simulink model "Islanding_case"  (R2024b)
settings: Solver=ode3  StartTime=0.0  StopTime=2.8  FixedStep=Ts  RelTol=1e-3  EnableMultiTasking=on
InitFcn:
  | Ts=100e-6;
  | Ts_Control=100e-6;
  | Ts_Power=100e-6;
  | tvv=0.1;
  | tr=1;
  | RelayEnableTime=1;
  | En_MC=1;
  | 
  | % ================= CHOOSE THE CASE HERE ==================
  | CaseNo    = 1;      % 1 = grid connected   2 = islanding   3 = fault during islanding
  | FaultType = 'none';   % 'none'  'LG'  'LL'  'LLG'  'LLL'  'LLLG'   (not used in case 2)
  | Qmismatch = 0;      % extra capacitive reactive power (% of 1.5 MW per load); try 1 in case 2 to see the inverter trip
  | % =========================================================
  | 
  | % ---- settings derived from the case (no need to edit)
  | switch CaseNo
  |     case 1, Tisland = 100; Pmismatch = 50; Tf = 2.0;   % grid + PV supply the load, fault at 2.0 s
  |     case 2, Tisland = 2.0; Pmismatch = 0;  Tf = 100;   % breakers open at 2.0 s, no fault
  |     case 3, Tisland = 2.0; Pmismatch = 0;  Tf = 2.3;   % breakers open at 2.0 s, fault at 2.3 s
  |     otherwise, error('CaseNo must be 1, 2 or 3');
  | end
  | FaultDur = 0.1;     % fault duration (s)
  | Tf_LG   = 100; Tf_LL = 100; Tf_LLG = 100; Tf_LLL = 100; Tf_LLLG = 100;   % 100 = never
  | switch upper(FaultType)
  |     case 'LG',   Tf_LG   = Tf;
  |     case 'LL',   Tf_LL   = Tf;
  |     case 'LLG',  Tf_LLG  = Tf;
  |     case 'LLL',  Tf_LLL  = Tf;
  |     case 'LLLG', Tf_LLLG = Tf;
  |     case 'NONE'
  |     otherwise, error('FaultType must be none, LG, LL, LLG, LLL or LLLG');
  | end
undefined symbols (not defined in the file or in its folder): DiscIntNeverNeededParam, Finit, Newton, Raphson, Tisland
libraries: simulink x33, spsOnDelayLib x17, powerlib_extras x11, eeGeneralControl x9, spsThreePhaseFaultLib x6, slpidlib x6, spsThreePhaseVIMeasurementLib x4, spsSampleandHoldLib x4, spsAlphaBetaZerotodq0Lib x4, spsThreePhaseSourceLib x4, spsThreePhaseBreakerLib x3, simulink_extras x3
(part 1 of 4)
settings Model: Creator=Administrator  LastModifiedBy=subas
settings SolverCC: AlgebraicLoopSolver=TrustRegion
settings DataIOCC: LimitDataPoints=on  SaveFormat=Array  SignalLoggingSaveFormat=ModelDataLogs  ReturnWorkspaceOutputs=off
settings OptimizationCC: ExpressionDepthLimit=2147483647  LifeSpan=inf
settings DebuggingCC: UnderspecifiedInitializationDetection=Classic  MergeDetectMultiDrivingBlocksExec=none  SolverPrmCheckMsg=warning  FcnCallInpInsideContextMsg=warning  UnconnectedInputMsg=warning  UnconnectedOutputMsg=warning  UnconnectedLineMsg=warning  StateNameClashWarn=warning  SFUnexpectedBacktrackingDiag=warning  SFNoUnconditionalDefaultTransitionDiag=warning  SFExecutionAtInitializationDiag=none  ArithmeticOperatorsInVariantConditions=warning
settings HardwareCC: ProdBitPerPointer=32  ProdBitPerSizeT=32  ProdBitPerPtrDiffT=32  ProdLargestAtomicFloat=None  ProdIntDivRoundTo=Undefined  ProdEndianess=Unspecified  ProdWordSize=32  ProdHWDeviceType=32-bit Generic
settings ModelReferenceCC: EnableRefExpFcnMdlSchedulingChecks=on  PropagateSignalLabelsOutOfModel=off
settings SFSimCC: SimUseLocalCustomCode=off  CustomCodeUndefinedFunction=UseInterfaceOnly
settings RTWCC: RTWUseLocalCustomCode=off  GPUComputeCapability=3.5
settings CodeAppCC: StateflowObjectComments=on
settings GRTTargetCC: TargetLangStandard=C89/C90 (ANSI)  CombineOutputUpdateFcns=off  GRTInterface=on
settings ConfigComp: CovMetricSettings=dw  CovSaveCumulativeToWorkspaceVar=on  CovSaveSingleToWorkspaceVar=on  CovExternalEMLEnable=off  CovSFcnEnable=off
settings SimscapeCC: SimscapeNormalizeSystem=off

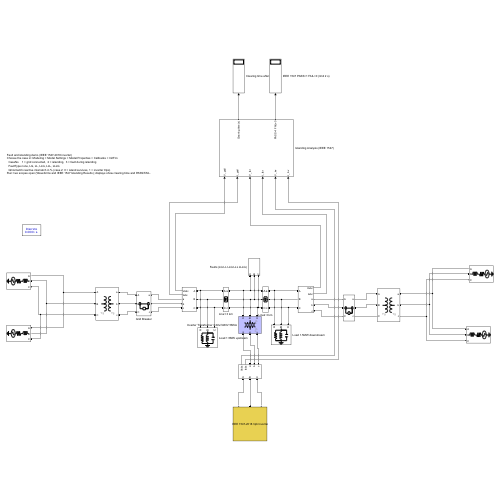
[thumbnail: Simulink's stored preview of the top-level diagram]
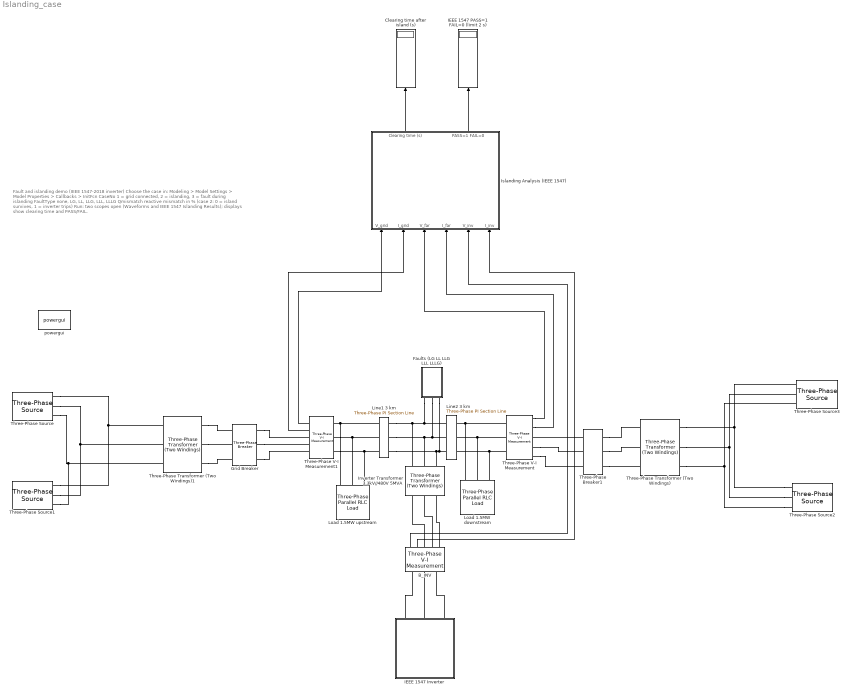
== system Islanding_case ==
  note: Fault and islanding demo (IEEE 1547-2018 inverter)
      | Choose the case in: Modeling > Model Settings > Model Properties > Callbacks > InitFcn
      |   CaseNo    1 = grid connected,  2 = islanding,  3 = fault during islanding
      |   FaultType none, LG, LL, LLG, LLL, LLLG
      |   Qmismatch reactive mismatch in % (case 2: 0 = island survives, 1 = inverter trips)
      | Run: two scopes open (Waveforms and IEEE 1547 Islanding Results); displays show clearing time and PASS/FAIL.
  B_INV : spsThreePhaseVIMeasurementLib/Three-Phase V-I Measurement  VoltageMeasurement=phase-to-ground  SetLabelV=off  LabelV=Vabc_PV  Vpu=off  VpuLL=off  CurrentMeasurement=yes  SetLabelI=off  LabelI=Iabc_PV  Ipu=off  Pbase=100e6  Vbase=500e3  OutputType=Complex  PhasorSimulation=off  PSBequivalent=0
  Clearing time after island (s) : Display
  Faults (LG LL LLG LLL LLLG) : Subsystem
  Grid Breaker : spsThreePhaseBreakerLib/Three-Phase Breaker  InitialState=closed  SwitchA=on  SwitchB=on  SwitchC=on  SwitchTimes=[Tisland]  External=off  BreakerResistance=0.001  SnubberResistance=1e6  SnubberCapacitance=inf  Measurements=None
  IEEE 1547 Inverter : Subsystem  mask(IEEE 1547-2018 Inverter){Pinv=1e6, N=3, RMSVnom=480/sqrt(3), NomFreq=50, Imax=1.2, Pref=1, EnableVW=0, En_VWatt=2, VWatt_V1=1.06, VWatt_V2=1.1, VWatt_P1=1, VWatt_P2=0, OLRT_VWatt=10, EnableFW=1, En_FW=2, dbOF=0.036, dbUF=0.036, KOF=0.05, KUF=0.05, Pmin=-1, OLRT_FW=5, EnableVQ=0, En_VVar=1, V1=0.92, V2=0.98, V3=1.02, V4=1.08, Q1=0.44, Q2=0, Q3=0, Q4=-0.44, OLRT_Vvar=5, QP_MODE_ENABLE=0, QP_CURVE_P1_GEN=0.2, QP_CURVE_P2_GEN=0.5, QP_CURVE_P3_GEN=1, QP_CURVE_Q1_GEN=0, QP_CURVE_Q2_GEN=0, QP_CURVE_Q3_GEN=-0.44, QP_CURVE_P1_ASP=-0.2, QP_CURVE_P2_ASP=-0.5, QP_CURVE_P3_ASP=-1, QP_CURVE_Q1_ASP=0, QP_CURVE_Q2_ASP=0, QP_CURVE_Q3_ASP=0.44, Constant_PF_Mode_Enable=0, Constant_PF=1, Constant_PF_Excitation=-1, CONST_Q_MODE_ENABLE=0, CONST_Q_ref=0, EnableMC=1, high_MC=1.2, low_MC=0.5, MC_recoveryrate=3, ES_V_HIGH=1.05, ES_V_LOW=0.917, ES_F_HIGH=50.1, ES_F_LOW=49.5, ES_DELAY=0, ES_RAMP_RATE=1, DVS_ENABLE=0, DVS_Threshold=0.88, Vref_DVS=1, Kpos=4, Kneg=4, EnableRMSOVProtection=1, OV2=1.2, OV2_time=0.16, OV1=1.1, OV1_time=13, UV1=0.88, UV1_time=21, UV2=0.5, UV2_time=2, EnableTOVProtection=1, EnableOFProtection=1, OF2=52, OF2_time=0.16, OF1=51.2, OF1_time=300, UF1=48.5, UF1_time=300, UF2=46.5, UF2_time=0.16, EnableOCProtection=1, OC2=2, OC2_time=0.16, OC1=1.5, OC1_time=0.5, GROUP2C_AI_ENABLE=1, GROUP2C_AI_DB=0.15, GROUP2C_AI_F_TH=2, GROUP2C_AI_LG1=0.1, GROUP2C_AI_LG2=0.2, GROUP2C_AI_HG1=0.2, GROUP2C_AI_HG2=0.2, GROUP2C_AI_LIMIT=0.5}
      mask prompts: Pinv "Inverter Apparent Power Rating (VA)"; N "Number of Inverters"; RMSVnom "Inverter Nominal RMS (l-g) Voltage (V)"; NomFreq "Nominal frequency (Hz)"; Imax "Maximum inverter current capacity (pu)"; Pref "Active Power reference (pu)"; EnableVW "Volt-Watt function Enable [Enable: 1; Disable: 0]"; En_VWatt "Enable Time Volt-Watt (sec)"; VWatt_V1 "VWatt curve point V1 setting (pu)"; VWatt_V2 "VWatt curve point V2 setting (pu)"; VWatt_P1 "VWatt curve point P1 setting (pu)"; VWatt_P2 "VWatt curve point P2 setting (pu)"; OLRT_VWatt "Open-Loop Response Time (sec)"; EnableFW "Freq-Watt function Enable [Enable: 1; Disable: 0]"; En_FW "Freq-Watt Enable Time (sec)"; dbOF "Over-freq deadband offset from nominal freq (Hz)"; dbUF "Under-freq deadband offset from nominal freq (Hz)"; KOF "Per unit over-freq change corresponding to a 1 pu power change"; KUF "Per unit under-freq change corresponding to a 1 pu power change"; Pmin "DER minimum active power (pu)"; OLRT_FW "Open-Loop Response Time (sec)"; EnableVQ "Volt-Var function Enable [Enable: 1; Disable: 0]"; En_VVar "Enable Time Volt-Var (sec)"; V1 "Voltage 1 (pu)"; V2 "Voltage 2 (pu)"; V3 "Voltage 3 (pu)"; V4 "Voltage 4 (pu)"; Q1 "Reactive Power 1 (pu)"; Q2 "Reactive Power 2 (pu)"; Q3 "Reactive Power 3 (pu)"; Q4 "Reactive Power 4 (pu)"; OLRT_Vvar "Open-Loop Response Time (sec)"; QP_MODE_ENABLE "Enable/Disable Watt-Var [Enable: 1; Diable: 0]"; QP_CURVE_P1_GEN "Watt-Var Curve Point P1 Setting (pu)"; QP_CURVE_P2_GEN "Watt-Var Curve Point P2 Setting (pu)"; QP_CURVE_P3_GEN "Watt-Var Curve Point P3 Setting (pu)"; QP_CURVE_Q1_GEN "Watt-Var Curve Point Q1 Setting (pu)"; QP_CURVE_Q2_GEN "Watt-Var Curve Point Q2 Setting (pu)"; QP_CURVE_Q3_GEN "Watt-Var Curve Point Q3 Setting (pu)"; QP_CURVE_P1_ASP "Watt-Var Curve Point P1' Setting (pu)"; QP_CURVE_P2_ASP "Watt-Var Curve Point P2' Setting (pu)"; QP_CURVE_P3_ASP "Watt-Var Curve Point P3' Setting (pu)"; QP_CURVE_Q1_ASP "Watt-Var Curve Point Q1' Setting (pu)"; QP_CURVE_Q2_ASP "Watt-Var Curve Point Q2' Setting (pu)"; QP_CURVE_Q3_ASP "Watt-Var Curve Point Q3' Setting (pu)"; Constant_PF_Mode_Enable "Enable/Disable Constant Power Factor [Enable: 1; Disable: 0]"; Constant_PF "Constant Power Factor Setting"; Constant_PF_Excitation "Constant Power Factor Excitation[Leading:1;Lagging:-1]"; CONST_Q_MODE_ENABLE "Enable/Disable Constant Reactive Power [Enable: 1; Disable: 0]"; CONST_Q_ref "Enter Reactive Power Reference Using the External Input [Injection:Positive;Absorption:Negative]"; EnableMC "Momentary Cessation Enable [Enable: 1; Disable: 0]"; high_MC "High-voltage momentary cessation threshold (pu)"; low_MC "Low-voltage momentary cessation threshold (pu)"; MC_recoveryrate "Momentary cessation recovery rate (pu/sec)"; ES_V_HIGH "Maximum applicable voltage to enter service (pu)"; ES_V_LOW "Minimum applicable voltage to enter service (pu)"; ES_F_HIGH "Maximum frequency to enter service (Hz)"; ES_F_LOW "Minimum frequency to enter service (Hz)"; ES_DELAY "Intentional delay before initiating soft-start (s)"; ES_RAMP_RATE "Enter active power ramp rate (pu/s)"; DVS_ENABLE "Enable/Disable DVS [Enable: 1; Disable: 0]"; DVS_Threshold "Voltage Threshold"; Vref_DVS "Pos seq Vref"; Kpos "Pos seq Kcomp"; Kneg "Neg seq Kcomp"; EnableRMSOVProtection "Enable/Disable RMS-based under- and over-voltage protection [Enable:1; Disable:0]"; OV2 "High voltage must trip OV2 voltage setting (pu)"; OV2_time "High voltage must trip OV2 duration setting (sec)"; OV1 "High voltage must trip OV1 voltage setting (pu)"; OV1_time "High voltage must trip OV1 duration setting (sec)"; UV1 "Low voltage must trip UV1 voltage setting (pu)"; UV1_time "Low voltage must trip UV1 duration setting (sec)"; UV2 "Low voltage must trip UV2 voltage setting (pu)"; UV2_time "Low voltage must trip UV2 duration setting (sec)"; EnableTOVProtection "Enable/Disable protection [Enable:1; Disable:0]"; EnableOFProtection "Enable/Disable under- and over-freqeuncy protection [Enable:1; Disable:0]"; OF2 "High freq must trip OF2 freq setting (Hz)"; OF2_time "High freq must trip OF2 duration setting (sec)"; OF1 "High freq must trip OF1 freq setting (Hz)"; OF1_time "High freq must trip OF1 duration setting (sec)"; UF1 "Low freq must trip UF1 freq setting (Hz)"; UF1_time "Low freq must trip UF1 duration setting (sec)"; UF2 "Low freq must trip UF2 freq setting (Hz)"; UF2_time "Low freq must trip UF2 duration setting (sec)"; EnableOCProtection "Enable/Disable under- and over-current protection [Enable:1; Disable:0]"; OC2 "Over-current must trip curve point OC2 current setting (pu)"; OC2_time "Over-current must trip curve point OC2 duration setting (s)"; OC1 "Over-current must trip curve point OC1 current setting (pu)"; OC1_time "Over-current must trip curve point OC1 duration setting (s)"; GROUP2C_AI_ENABLE "Enable/Disable Active Islanding Detection [Enable: 1; Disable: 0]"; GROUP2C_AI_DB "Dead-Band (No perturbations within deadband)"; GROUP2C_AI_F_TH "Frequency Threshold (Hz)"; GROUP2C_AI_LG1 "Low frequency gain 1"; GROUP2C_AI_LG2 "Low frequency gain 2"; GROUP2C_AI_HG1 "High frequency gain 1"; GROUP2C_AI_HG2 "High frequency gain 2"; GROUP2C_AI_LIMIT "Limit on reactive power perturbations (pu)"
      mask help:
      | Note:
      |  1) The active power rating (Watt) and the apparent power rating (VA) are the same for this inverter
      |  2) Any disturbances (fault, etc.) should be applied after the startup process has completed and a steady state has been reached
      |  3) Make sure ONLY ONE Reactive Power Support Function is activated (Volt-Var, Constant PF, Constant Q, or Watt-Var)
      |  4) Enable times for Volt-Watt, Volt-Var, and Freq-Watt functions are not inverter settings but provided to allow a user to simulate the impact of activating these functions
      |  5) When representing a battery or PV plus battery inverter:
      |    a) The active power reference should be set to a negative value (between -1pu and 0) if the inverter is in charging mode
      |    b) The Volt-Watt curve point P2 and the Freq-Watt DER minimum active power settings can be set to negative values between -1pu and 0
      mask DialogControl ParameterTabVar01 Prompt: Physical Elements
      mask DialogControl Container17 Prompt: Control Elements
      mask DialogControl Container31 Prompt: Active Power Support Functions
      mask DialogControl Container54 Prompt: 1. Voltage-Active Power (Volt-Watt) Function
      mask DialogControl Container32 Prompt: 2. Frequency - Active Power (Frequency-Watt) Function
      mask DialogControl Container37 Prompt: Reactive Power Support Functions
      mask DialogControl Container38 Prompt: 1. Voltage-Reactive Power (Volt-Var) Function
      mask DialogControl Container40 Prompt: 2. Active Power-Reactive Power (Watt - Var) Function
      mask DialogControl Container42 Prompt: 3. Constant Power Factor Function
      mask DialogControl Container44 Prompt: 4. Constant Reactive Power Mode
      mask DialogControl Container46 Prompt: Momentary Cessation
      mask DialogControl Container48 Prompt: Enter Service Criteria
      mask DialogControl Container53 Prompt: Dynamic Voltage Support
      mask DialogControl Container26 Prompt: Protection Elements
      mask DialogControl Container20 Prompt: Under- and Over-voltage protection
      mask DialogControl Container56 Prompt: Transient Over-Voltage Protection
      mask DialogControl Container22 Prompt: Under-and Over-frequency protection
      mask DialogControl Container24 Prompt: Over Current Protection
      mask DialogControl Container50 Prompt: Active Islanding Detection
      mask Display: disp('IEEE 1547-2018 3ph Inverter')
  IEEE 1547 PASS=1 FAIL=0 (limit 2 s) : Display
  Inverter Transformer 3.3kV//480V 5MVA : spsThreePhaseTransformerTwoWindingsLib/Three-Phase Transformer (Two Windings)  Winding1Connection=Yg  Winding2Connection=Yg  CoreType=Three single-phase transformers  SetSaturation=off  Hysteresis=off  DataFile='basic_model'  SetInitialFlux=off  Measurements=None  UNITS=pu  NominalPower=[5e6 50]  Winding1="[ 3.3e3  0.025/10   0.025 ]"  Winding2="[ 480  0.025/10  0.025]"  Rm=500  Lm=500  L0=0.5  Saturation="[ 0,0  ;  0.005,1.2  ;  1.0,1.4 ]"  InitialFluxes=[ 0.8 , -0.8 , 0.7 ]  BreakLoop=off  DiscreteSolver=Trapezoidal iterative  DataType=off  TransfoNumber=0
  Islanding Analysis (IEEE 1547) : Subsystem
  Line1 3 km : spsThreePhasePISectionLineLib/Three-Phase PI Section Line  LConnTagsString=a|b|c  RConnTagsString=A|B|C  Length=3  Frequency=50  Resistances=[0.0132 0.132]  Inductances=[0.9337e-3 4.1264e-3]  Capacitances=[12.74e-9 7.751e-9]
  Line2 3 km : spsThreePhasePISectionLineLib/Three-Phase PI Section Line  LConnTagsString=a|b|c  RConnTagsString=A|B|C  Length=3  Frequency=50  Resistances=[0.0132 0.132]  Inductances=[0.9337e-3 4.1264e-3]  Capacitances=[12.74e-9 7.751e-9]
  Load 1.5MW downstream : spsThreePhaseParallelRLCLoadLib/Three-Phase Parallel RLC Load  LConnTagsString=A|B|C  Configuration=Y (grounded)  NominalVoltage=3.3e3  Vabc=[1e3 1e3 1e3]  Vabcp=[1e3 1e3 1e3]  NominalFrequency=50  UnbalancedPower=off  ActivePower=1.48367e+06*(1+Pmismatch/100)  InductivePower=1.37206e+06  CapacitivePower=1.60436e+06+Qmismatch/100*1.5e6  Pabc=[10e3 9e3 11e3]  QLabc=[100 90 110]  QCabc=[100 90 110]  Pabcp=[10e3 9e3 11e3]  QLabcp=[100 90 110]  QCabcp=[100 90 110]  Measurements=None  LoadType=constant Z
  Load 1.5MW upstream : spsThreePhaseParallelRLCLoadLib/Three-Phase Parallel RLC Load  LConnTagsString=A|B|C  Configuration=Y (grounded)  NominalVoltage=3.3e3  Vabc=[1e3 1e3 1e3]  Vabcp=[1e3 1e3 1e3]  NominalFrequency=50  UnbalancedPower=off  ActivePower=1.48335e+06*(1+Pmismatch/100)  InductivePower=1.37193e+06  CapacitivePower=1.60383e+06+Qmismatch/100*1.5e6  Pabc=[10e3 9e3 11e3]  QLabc=[100 90 110]  QCabc=[100 90 110]  Pabcp=[10e3 9e3 11e3]  QLabcp=[100 90 110]  QCabcp=[100 90 110]  Measurements=None  LoadType=constant Z
  Three-Phase Transformer (Two Windings)1 : spsThreePhaseTransformerTwoWindingsLib/Three-Phase Transformer (Two Windings)  Winding1Connection=Yg  Winding2Connection=Yg  CoreType=Three single-phase transformers  SetSaturation=off  Hysteresis=off  DataFile='hysteresis'  SetInitialFlux=off  Measurements=None  UNITS=pu  NominalPower=[ 250e6 , 50 ]  Winding1=[132e3 , 0.002 , 0.08 ]  Winding2=[3.3e3 , 0.002 , 0.08 ]  Rm=500  Lm=500  L0=0.5  Saturation=[ 0,0 ; 0.0024,1.2 ; 1.0,1.52 ]  InitialFluxes=[ 0.8 , -0.8 , 0.7 ]  BreakLoop=off  DiscreteSolver=Trapezoidal iterative  DataType=off  TransfoNumber=1
  Three-Phase V-I Measurement : spsThreePhaseVIMeasurementLib/Three-Phase V-I Measurement  VoltageMeasurement=phase-to-ground  SetLabelV=off  LabelV=Vabc  Vpu=off  VpuLL=off  CurrentMeasurement=yes  SetLabelI=off  LabelI=Iabc  Ipu=off  Pbase=100e6  Vbase=500e3  OutputType=Complex  PhasorSimulation=off  PSBequivalent=0
  Three-Phase V-I Measurement1 : spsThreePhaseVIMeasurementLib/Three-Phase V-I Measurement  VoltageMeasurement=phase-to-ground  SetLabelV=off  LabelV=Vabc  Vpu=off  VpuLL=off  CurrentMeasurement=yes  SetLabelI=off  LabelI=Iabc  Ipu=off  Pbase=100e6  Vbase=500e3  OutputType=Complex  PhasorSimulation=off  PSBequivalent=0
  Three-Phase Breaker1 : spsThreePhaseBreakerLib/Three-Phase Breaker  InitialState=closed  SwitchA=on  SwitchB=on  SwitchC=on  SwitchTimes=[Tisland]  External=off  BreakerResistance=0.001  SnubberResistance=1e6  SnubberCapacitance=inf  Measurements=None
  Three-Phase Source : spsThreePhaseSourceLib/Three-Phase Source  InternalConnection=Yg  VoltagePhases=off  Voltage=132e3  PhaseAngle=0  Voltage_phases=[25e3 25e3 25e3]/sqrt(3)  PhaseAngles_phases=[0 -120 +120]  Frequency=50  NonIdealSource=on  SpecifyImpedance=off  Resistance=12  Inductance=16.58e-3  ShortCircuitLevel=50e6  BaseVoltage=11e3  XRratio=7  BusType=PV  Pref=50e6  Qref=0  Prefabc=[10e3, 10e3, 10e3]  Qrefabc=[0, 0, 0]  Qmin=-inf  Qmax=inf
  Three-Phase Source1 : spsThreePhaseSourceLib/Three-Phase Source  InternalConnection=Yg  VoltagePhases=off  Voltage=132e3  PhaseAngle=0  Voltage_phases=[25e3 25e3 25e3]/sqrt(3)  PhaseAngles_phases=[0 -120 +120]  Frequency=50  NonIdealSource=on  SpecifyImpedance=off  Resistance=12  Inductance=16.58e-3  ShortCircuitLevel=50e6  BaseVoltage=11e3  XRratio=7  BusType=PV  Pref=50e6  Qref=0  Prefabc=[10e3, 10e3, 10e3]  Qrefabc=[0, 0, 0]  Qmin=-inf  Qmax=inf
  Three-Phase Source2 : spsThreePhaseSourceLib/Three-Phase Source  InternalConnection=Yg  VoltagePhases=off  Voltage=132e3  PhaseAngle=0  Voltage_phases=[25e3 25e3 25e3]/sqrt(3)  PhaseAngles_phases=[0 -120 +120]  Frequency=50  NonIdealSource=on  SpecifyImpedance=off  Resistance=8.4  Inductance=16.58e-3  ShortCircuitLevel=20e6  BaseVoltage=11e3  XRratio=7  BusType=PV  Pref=20e6  Qref=0  Prefabc=[10e3, 10e3, 10e3]  Qrefabc=[0, 0, 0]  Qmin=-inf  Qmax=inf
  Three-Phase Source3 : spsThreePhaseSourceLib/Three-Phase Source  InternalConnection=Yg  VoltagePhases=off  Voltage=132e3  PhaseAngle=0  Voltage_phases=[25e3 25e3 25e3]/sqrt(3)  PhaseAngles_phases=[0 -120 +120]  Frequency=50  NonIdealSource=on  SpecifyImpedance=off  Resistance=12  Inductance=16.58e-3  ShortCircuitLevel=50e6  BaseVoltage=11e3  XRratio=7  BusType=PV  Pref=50e6  Qref=0  Prefabc=[10e3, 10e3, 10e3]  Qrefabc=[0, 0, 0]  Qmin=-inf  Qmax=inf
  Three-Phase Transformer (Two Windings) : spsThreePhaseTransformerTwoWindingsLib/Three-Phase Transformer (Two Windings)  Winding1Connection=Yg  Winding2Connection=Yg  CoreType=Three single-phase transformers  SetSaturation=off  Hysteresis=off  DataFile='hysteresis'  SetInitialFlux=off  Measurements=None  UNITS=pu  NominalPower=[ 250e6 , 50 ]  Winding1=[3.3e3 , 0.002 , 0.08 ]  Winding2=[132e3 , 0.002 , 0.08 ]  Rm=500  Lm=500  L0=0.5  Saturation=[ 0,0 ; 0.0024,1.2 ; 1.0,1.52 ]  InitialFluxes=[ 0.8 , -0.8 , 0.7 ]  BreakLoop=off  DiscreteSolver=Trapezoidal iterative  DataType=off  TransfoNumber=1
  powergui : spspowerguiLib/powergui  Priority=1  SimulationMode=Discrete  SampleTime=Ts  frequency=50  Iterations=50  frequencyindice=50  Pbase=100e6  ErrMax=1e-4  UnitsV=kV  UnitsW=MW  buscounter=0  FunctionMessages=off  echomessages=off  EnableUseOfTLC=off  CurrentSourceSwitches=off  DisableSnubberDevices=off  DisableRonSwitches=off  DisableVfSwitches=off  DisplayEquations=off  AutomaticDiscreteSolvers=off  SolverType=Tustin  Interpol=off  ExternalGateDelay=off  methode=off  Ts=0  x0status=blocks  SPID=off  SwTol=0  HookPort=off  NonlinearTolerance=1e-4  nMaxIteration=100  ContinueOnMaxIteration=off  RestoreLinks=warning  ResistiveCurrentMeasurement=off  Frange=[0:2:500]  Ylog=off  Xlog=on  ShowGrid=off  save=off  variable=ZData  structure=0  ZoomFFT=off  StartTime=0.0  cycles=1  DisplayStyle=1  fundamental=60  FreqAxis=off  MaxFrequency=1000  frequencyindicesteady=1  RmsSteady=1  display=off
  wires:
  Three-Phase V-I Measurement1/1 -> Islanding Analysis (IEEE 1547)/1(V_grid)
  Three-Phase V-I Measurement1/2 -> Islanding Analysis (IEEE 1547)/2(I_grid)
  Three-Phase V-I Measurement/1 -> Islanding Analysis (IEEE 1547)/3(V_far)
  Three-Phase V-I Measurement/2 -> Islanding Analysis (IEEE 1547)/4(I_far)
  B_INV/1 -> Islanding Analysis (IEEE 1547)/5(V_inv)
  B_INV/2 -> Islanding Analysis (IEEE 1547)/6(I_inv)
  Islanding Analysis (IEEE 1547)/1(Clearing time (s)) -> Clearing time after island (s)/1
  Islanding Analysis (IEEE 1547)/2(PASS=1 FAIL=0) -> IEEE 1547 PASS=1 FAIL=0 (limit 2 s)/1
  connections:
  Line1 3 km/RConn1 -- Inverter Transformer 3.3kV//480V 5MVA/LConn1 -- Faults (LG LL LLG LLL LLLG)/LConn1 -- Line2 3 km/LConn1
  Line1 3 km/RConn3 -- Inverter Transformer 3.3kV//480V 5MVA/LConn3 -- Faults (LG LL LLG LLL LLLG)/LConn3 -- Line2 3 km/LConn3
  Line1 3 km/RConn2 -- Inverter Transformer 3.3kV//480V 5MVA/LConn2 -- Faults (LG LL LLG LLL LLLG)/LConn2 -- Line2 3 km/LConn2
  Three-Phase Source/RConn1 -- Three-Phase Source1/RConn1 -- Three-Phase Transformer (Two Windings)1/LConn1
  Three-Phase Source/RConn2 -- Three-Phase Source1/RConn2 -- Three-Phase Transformer (Two Windings)1/LConn2
  Three-Phase Source/RConn3 -- Three-Phase Source1/RConn3 -- Three-Phase Transformer (Two Windings)1/LConn3
  Three-Phase V-I Measurement1/LConn1 -- Line1 3 km/LConn1 -- Load 1.5MW upstream/LConn1
  Three-Phase V-I Measurement1/LConn2 -- Line1 3 km/LConn2 -- Load 1.5MW upstream/LConn2
  Three-Phase V-I Measurement1/LConn3 -- Line1 3 km/LConn3 -- Load 1.5MW upstream/LConn3
  Line2 3 km/RConn1 -- Three-Phase V-I Measurement/LConn1 -- Load 1.5MW downstream/LConn1
  Line2 3 km/RConn2 -- Three-Phase V-I Measurement/LConn2 -- Load 1.5MW downstream/LConn2
  Line2 3 km/RConn3 -- Three-Phase V-I Measurement/LConn3 -- Load 1.5MW downstream/LConn3
  IEEE 1547 Inverter/LConn1 -- B_INV/LConn1
  B_INV/RConn1 -- Inverter Transformer 3.3kV//480V 5MVA/RConn1
  IEEE 1547 Inverter/LConn2 -- B_INV/LConn2
  B_INV/RConn2 -- Inverter Transformer 3.3kV//480V 5MVA/RConn2
  IEEE 1547 Inverter/LConn3 -- B_INV/LConn3
  B_INV/RConn3 -- Inverter Transformer 3.3kV//480V 5MVA/RConn3
  Three-Phase Source2/RConn1 -- Three-Phase Transformer (Two Windings)/RConn1 -- Three-Phase Source3/RConn1
  Three-Phase Source2/RConn2 -- Three-Phase Transformer (Two Windings)/RConn2 -- Three-Phase Source3/RConn2
  Three-Phase Source2/RConn3 -- Three-Phase Transformer (Two Windings)/RConn3 -- Three-Phase Source3/RConn3
  Three-Phase Transformer (Two Windings)1/RConn1 -- Grid Breaker/LConn1
  Grid Breaker/RConn1 -- Three-Phase V-I Measurement1/RConn1
  Three-Phase Transformer (Two Windings)1/RConn2 -- Grid Breaker/LConn2
  Grid Breaker/RConn2 -- Three-Phase V-I Measurement1/RConn2
  Three-Phase Transformer (Two Windings)1/RConn3 -- Grid Breaker/LConn3
  Grid Breaker/RConn3 -- Three-Phase V-I Measurement1/RConn3
  Three-Phase Breaker1/LConn1 -- Three-Phase V-I Measurement/RConn1
  Three-Phase Breaker1/RConn1 -- Three-Phase Transformer (Two Windings)/LConn1
  Three-Phase V-I Measurement/RConn2 -- Three-Phase Breaker1/LConn2
  Three-Phase Breaker1/RConn2 -- Three-Phase Transformer (Two Windings)/LConn2
  Three-Phase V-I Measurement/RConn3 -- Three-Phase Breaker1/LConn3
  Three-Phase Breaker1/RConn3 -- Three-Phase Transformer (Two Windings)/LConn3

== system Islanding_case/Faults (LG LL LLG LLL LLLG) ==
  Three-Phase Fault1 : spsThreePhaseFaultLib/Three-Phase Fault  InitialStates=0  FaultA=on  FaultB=on  FaultC=off  GroundFault=on  SwitchTimes=[Tf_LLG Tf_LLG+FaultDur]  External=off  SwitchStatus=NaN  FaultResistance=0.001  GroundResistance=0.001  SnubberResistance=1e6  SnubberCapacitance=inf  Measurements=None
  Three-Phase Fault2 : spsThreePhaseFaultLib/Three-Phase Fault  InitialStates=0  FaultA=on  FaultB=off  FaultC=off  GroundFault=on  SwitchTimes=[Tf_LG Tf_LG+FaultDur]  External=off  SwitchStatus=NaN  FaultResistance=0.001  GroundResistance=0.001  SnubberResistance=1e6  SnubberCapacitance=inf  Measurements=None
  Three-Phase Fault3 : spsThreePhaseFaultLib/Three-Phase Fault  InitialStates=0  FaultA=off  FaultB=on  FaultC=on  GroundFault=off  SwitchTimes=[Tf_LL Tf_LL+FaultDur]  External=off  SwitchStatus=NaN  FaultResistance=0.001  GroundResistance=0.001  SnubberResistance=1e6  SnubberCapacitance=inf  Measurements=None
  Three-Phase Fault4 : spsThreePhaseFaultLib/Three-Phase Fault  InitialStates=0  FaultA=on  FaultB=on  FaultC=on  GroundFault=on  SwitchTimes=[Tf_LLLG Tf_LLLG+FaultDur]  External=off  SwitchStatus=NaN  FaultResistance=0.001  GroundResistance=0.001  SnubberResistance=1e6  SnubberCapacitance=inf  Measurements=None
  Three-Phase Fault5 : spsThreePhaseFaultLib/Three-Phase Fault  InitialStates=0  FaultA=on  FaultB=on  FaultC=on  GroundFault=off  SwitchTimes=[Tf_LLL Tf_LLL+FaultDur]  External=off  SwitchStatus=NaN  FaultResistance=0.001  GroundResistance=0.001  SnubberResistance=1e6  SnubberCapacitance=inf  Measurements=None
  Three-Phase Fault6 : spsThreePhaseFaultLib/Three-Phase Fault  InitialStates=0  FaultA=off  FaultB=off  FaultC=off  GroundFault=off  SwitchTimes=[100 100.05]  External=off  SwitchStatus=NaN  FaultResistance=0.001  GroundResistance=0.001  SnubberResistance=1e6  SnubberCapacitance=inf  Measurements=None
  A : PMIOPort  Side=Left
  B : PMIOPort  Port=2  Side=Left
  C : PMIOPort  Port=3  Side=Left
  connections:
  Three-Phase Fault2/LConn2 -- Three-Phase Fault6/LConn2 -- Three-Phase Fault4/LConn2 -- Three-Phase Fault5/LConn2 -- Three-Phase Fault3/LConn2 -- Three-Phase Fault1/LConn2 -- B/RConn1
  Three-Phase Fault2/LConn3 -- Three-Phase Fault6/LConn3 -- Three-Phase Fault4/LConn3 -- Three-Phase Fault5/LConn3 -- Three-Phase Fault3/LConn3 -- Three-Phase Fault1/LConn3 -- C/RConn1
  Three-Phase Fault2/LConn1 -- Three-Phase Fault6/LConn1 -- Three-Phase Fault4/LConn1 -- Three-Phase Fault5/LConn1 -- Three-Phase Fault3/LConn1 -- Three-Phase Fault1/LConn1 -- A/RConn1

== system Islanding_case/IEEE 1547 Inverter ==
  " Inverter Hardware" : Subsystem
  DC Voltage Source : spsDCVoltageSourceLib/DC Voltage Source  Amplitude=RMSVnom*sqrt(3)*2.5  Measurements=None
  "Inverter measurements, controls, and protection" : Subsystem
  A : PMIOPort  Tag=PMCPort  Side=Left
  B : PMIOPort  Tag=PMCPort  Port=2  Side=Left
  C : PMIOPort  Tag=PMCPort  Port=3  Side=Left
  wires:
  [AC_Brk_Ctrl] -> " Inverter Hardware"/2(AC_Brk_Ctrl)
  [Uref] -> " Inverter Hardware"/1(Uref)
  [VPCC] -> "Inverter measurements, controls, and protection"/1(VPCC_inv)
  "Inverter measurements, controls, and protection"/1(Uref) -> [Uref]
  "Inverter measurements, controls, and protection"/2(AC Brk Ctrl) -> [AC_Brk_Ctrl]
  [IPCC] -> "Inverter measurements, controls, and protection"/2(IPCC)
  " Inverter Hardware"/2(IPCC) -> [IPCC]
  " Inverter Hardware"/1(VPCC) -> [VPCC]
  connections:
  DC Voltage Source/LConn1 -- " Inverter Hardware"/LConn2
  DC Voltage Source/RConn1 -- " Inverter Hardware"/LConn1
  " Inverter Hardware"/RConn3 -- C/RConn1
  " Inverter Hardware"/RConn2 -- B/RConn1
  " Inverter Hardware"/RConn1 -- A/RConn1

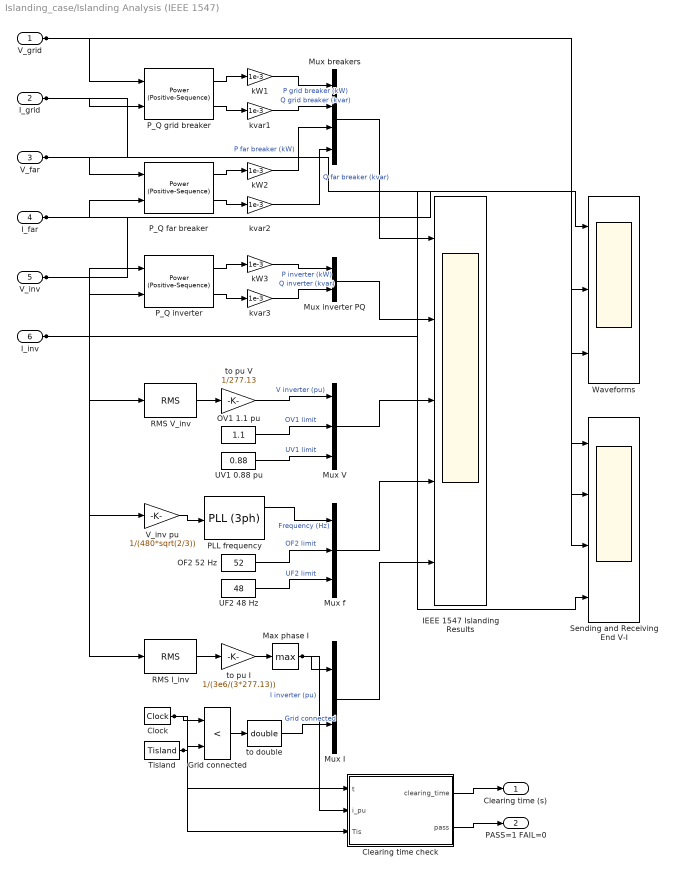
== system Islanding_case/Islanding Analysis (IEEE 1547) ==
  V_grid : Inport
  I_grid : Inport  Port=2
  V_far : Inport  Port=3
  I_far : Inport  Port=4
  V_inv : Inport  Port=5
  I_inv : Inport  Port=6
  Clearing time check : MATLAB Function  TreatAsAtomicUnit=on
  Clock : DigitalClock  SampleTime=Ts
  Grid connected : RelationalOperator  Operator=<  OutDataTypeStr=boolean  RndMeth=Simplest  InputSameDT=off
  IEEE 1547 Islanding Results : Scope  NumInputPorts=5
  Max phase I : MinMax  Function=max
  Mux I : Mux  Inputs=2
  Mux V : Mux  Inputs=3
  Mux breakers : Mux
  Mux f : Mux  Inputs=3
  Mux inverter PQ : Mux  Inputs=2
  OF2 52 Hz : Constant  Value=52  SampleTime=Ts
  OV1 1.1 pu : Constant  Value=1.1  SampleTime=Ts
  PLL frequency : spsPLL3phLib/PLL (3ph)  Fmin=40  Par_Init=[0, 50]  ParK=[180, 3200, 1]  TcD=1e-4  MaxRateChangeFreq=200  FilterCutOffFreq=25  Ts=Ts  AGC=on
  P_Q far breaker : spsPowerPositiveSequenceLib/Power (Positive-Sequence)  Freq=50  Vinit=[0, 0]  Iinit=[0, 0]  Ts=Ts
  P_Q grid breaker : spsPowerPositiveSequenceLib/Power (Positive-Sequence)  Freq=50  Vinit=[0, 0]  Iinit=[0, 0]  Ts=Ts
  P_Q inverter : spsPowerPositiveSequenceLib/Power (Positive-Sequence)  Freq=50  Vinit=[0, 0]  Iinit=[0, 0]  Ts=Ts
  RMS I_inv : spsRMSLib/RMS  TrueRMS=on  Freq=50  RMSInit=0  Ts=Ts
  RMS V_inv : spsRMSLib/RMS  TrueRMS=on  Freq=50  RMSInit=277.13  Ts=Ts
  Sending and Receiving End V-I : Scope  NumInputPorts=4
  Tisland : Constant  Value=Tisland  SampleTime=Ts
  UF2 48 Hz : Constant  Value=48  SampleTime=Ts
  UV1 0.88 pu : Constant  Value=0.88  SampleTime=Ts
  V_inv pu : Gain  Gain=1/(480*sqrt(2/3))
  Waveforms : Scope  NumInputPorts=3
  kW1 : Gain  Gain=1e-3
  kW2 : Gain  Gain=1e-3
  kW3 : Gain  Gain=1e-3
  kvar1 : Gain  Gain=1e-3
  kvar2 : Gain  Gain=1e-3
  kvar3 : Gain  Gain=1e-3
  to double : DataTypeConversion  OutDataTypeStr=double  SaturateOnIntegerOverflow=off  RndMeth=Floor
  to pu I : Gain  Gain=1/(3e6/(3*277.13))
  to pu V : Gain  Gain=1/277.13
  Clearing time (s) : Outport
  PASS=1 FAIL=0 : Outport  Port=2
  wires:
  V_grid/1 -> P_Q grid breaker/1, Sending and Receiving End V-I/1
  I_grid/1 -> P_Q grid breaker/2, Waveforms/1, Sending and Receiving End V-I/2
  P_Q grid breaker/1 -> kW1/1
  P_Q grid breaker/2 -> kvar1/1
  V_far/1 -> P_Q far breaker/1, Sending and Receiving End V-I/3
  I_far/1 -> P_Q far breaker/2, Sending and Receiving End V-I/4
  P_Q far breaker/1 -> kW2/1
  P_Q far breaker/2 -> kvar2/1
  V_inv/1 -> P_Q inverter/1, RMS V_inv/1, V_inv pu/1, Waveforms/3
  I_inv/1 -> P_Q inverter/2, RMS I_inv/1, Waveforms/2
  P_Q inverter/1 -> kW3/1
  P_Q inverter/2 -> kvar3/1
  kW1/1 -> Mux breakers/1  "P grid breaker (kW)"
  kvar1/1 -> Mux breakers/2  "Q grid breaker (kvar)"
  kW2/1 -> Mux breakers/3  "P far breaker (kW)"
  kvar2/1 -> Mux breakers/4  "Q far breaker (kvar)"
  kW3/1 -> Mux inverter PQ/1  "P inverter (kW)"
  kvar3/1 -> Mux inverter PQ/2  "Q inverter (kvar)"
  RMS V_inv/1 -> to pu V/1
  to pu V/1 -> Mux V/1  "V inverter (pu)"
  OV1 1.1 pu/1 -> Mux V/2  "OV1 limit"
  UV1 0.88 pu/1 -> Mux V/3  "UV1 limit"
  V_inv pu/1 -> PLL frequency/1
  PLL frequency/1 -> Mux f/1  "Frequency (Hz)"
  OF2 52 Hz/1 -> Mux f/2  "OF2 limit"
  UF2 48 Hz/1 -> Mux f/3  "UF2 limit"
  RMS I_inv/1 -> to pu I/1
  to pu I/1 -> Max phase I/1
  Clock/1 -> Grid connected/1, Clearing time check/1(t)
  Tisland/1 -> Grid connected/2, Clearing time check/3(Tis)
  Grid connected/1 -> to double/1
  Max phase I/1 -> Mux I/1, Clearing time check/2(i_pu)  "I inverter (pu)"
  to double/1 -> Mux I/2  "Grid connected"
  Clearing time check/1(clearing_time) -> Clearing time (s)/1
  Clearing time check/2(pass) -> PASS=1 FAIL=0/1
  Mux breakers/1 -> IEEE 1547 Islanding Results/1
  Mux inverter PQ/1 -> IEEE 1547 Islanding Results/2
  Mux V/1 -> IEEE 1547 Islanding Results/3
  Mux f/1 -> IEEE 1547 Islanding Results/4
  Mux I/1 -> IEEE 1547 Islanding Results/5

== system Islanding_case/IEEE 1547 Inverter/ Inverter Hardware ==
  note: AC filter inductor
  note: AC filter capacitor
  note: AC side Breaker is controlled in controller subsystem
  Uref : Inport
  AC_Brk_Ctrl : Inport  Port=2
  Breaker : spsThreePhaseBreakerLib/Three-Phase Breaker  InitialState=closed  SwitchA=on  SwitchB=on  SwitchC=on  SwitchTimes="[4/NomFreq  10/NomFreq]"  External=on  BreakerResistance=1e-9  SnubberResistance=1e6  SnubberCapacitance=inf  Measurements=None
      link override Breaker A: SwitchingTimes="[ 1/NomFreq  5/NomFreq ]"
      link override Breaker B: SwitchingTimes="[ 1/NomFreq  5/NomFreq ]"
      link override Breaker C: SwitchingTimes="[ 1/NomFreq  5/NomFreq ]"
  C_f : spsThreePhaseParallelRLCBranchLib/Three-Phase Parallel RLC Branch  LConnTagsString=A|B|C  RConnTagsString=A|B|C  BranchType=RC  Resistance=0.3  Inductance=1e-3  Capacitance=(445e-6)*(N*Pinv/2.2e6)/(RMSVnom*sqrt(3)/385)^2  Measurements=None
  L_f : spsThreePhaseSeriesRLCBranchLib/Three-Phase Series RLC Branch  LConnTagsString=A|B|C  RConnTagsString=A|B|C  BranchType=RL  Resistance=(0.01e-3)*(RMSVnom*sqrt(3)/385)^2/(N*Pinv/2.2e6)  Inductance=(48e-6)*(RMSVnom*sqrt(3)/385)^2/(N*Pinv/2.2e6)  Capacitance=1.0  Measurements=None
  PWM Average model : spsUniversalBridgeLib/Universal Bridge  Arms=3  SnubberResistance=5000  SnubberCapacitance=inf  Device=Average-model based VSC  Ron=1e-3  Lon=0  ForwardVoltages="[  1  1  ]"  ForwardVoltage=.8  GTOparameters=[ 1e-6 ,1e-6 ]  IGBTparameters=[ 1e-6 , 2e-6 ]  Measurements=None  Measurements_2=None  converterType=Rectifier
      link override "Model/discrete IGBT/g1,d1,g2,d2, ...": NumberOfDimensions=1
      settings: AttributesFormatString=\n
  Three-Phase V-I Measurement8 : spsThreePhaseVIMeasurementLib/Three-Phase V-I Measurement  VoltageMeasurement=phase-to-ground  SetLabelV=off  LabelV=Vabc  Vpu=off  VpuLL=off  CurrentMeasurement=yes  SetLabelI=off  LabelI=Iabc  Ipu=off  Pbase=100e6  Vbase=500e3  OutputType=Complex  PhasorSimulation=off  PSBequivalent=0
  DC+ : PMIOPort  Side=Left
  DC- : PMIOPort  Port=2  Side=Left
  A : PMIOPort  Tag=PMCPort  Port=3  Side=Right
  B : PMIOPort  Tag=PMCPort  Port=4  Side=Right
  C : PMIOPort  Tag=PMCPort  Port=5  Side=Right
  VPCC : Outport  VectorParamsAs1DForOutWhenUnconnected=off
  IPCC : Outport  Port=2  VectorParamsAs1DForOutWhenUnconnected=off
  wires:
  Three-Phase V-I Measurement8/1 -> [VPCC]
  Three-Phase V-I Measurement8/2 -> [IPCC]
  [AC_Brk_Ctrl] -> Breaker/1
  AC_Brk_Ctrl/1 -> [AC_Brk_Ctrl]
  [IPCC] -> IPCC/1
  [VPCC] -> VPCC/1
  Uref/1 -> [Uref]
  [Uref] -> PWM Average model/1
  connections:
  L_f/LConn3 -- PWM Average model/LConn3
  L_f/LConn1 -- PWM Average model/LConn1
  L_f/LConn2 -- PWM Average model/LConn2
  PWM Average model/RConn2 -- DC-/RConn1
  PWM Average model/RConn1 -- DC+/RConn1
  C_f/RConn1 -- C_f/LConn3 -- Breaker/LConn1 -- L_f/RConn1
  Three-Phase V-I Measurement8/LConn1 -- Breaker/RConn1
  Three-Phase V-I Measurement8/LConn2 -- Breaker/RConn2
  Three-Phase V-I Measurement8/LConn3 -- Breaker/RConn3
  Three-Phase V-I Measurement8/RConn1 -- A/RConn1
  Three-Phase V-I Measurement8/RConn2 -- B/RConn1
  Three-Phase V-I Measurement8/RConn3 -- C/RConn1
  C_f/RConn3 -- C_f/LConn2 -- Breaker/LConn3 -- L_f/RConn3
  C_f/RConn2 -- C_f/LConn1 -- Breaker/LConn2 -- L_f/RConn2

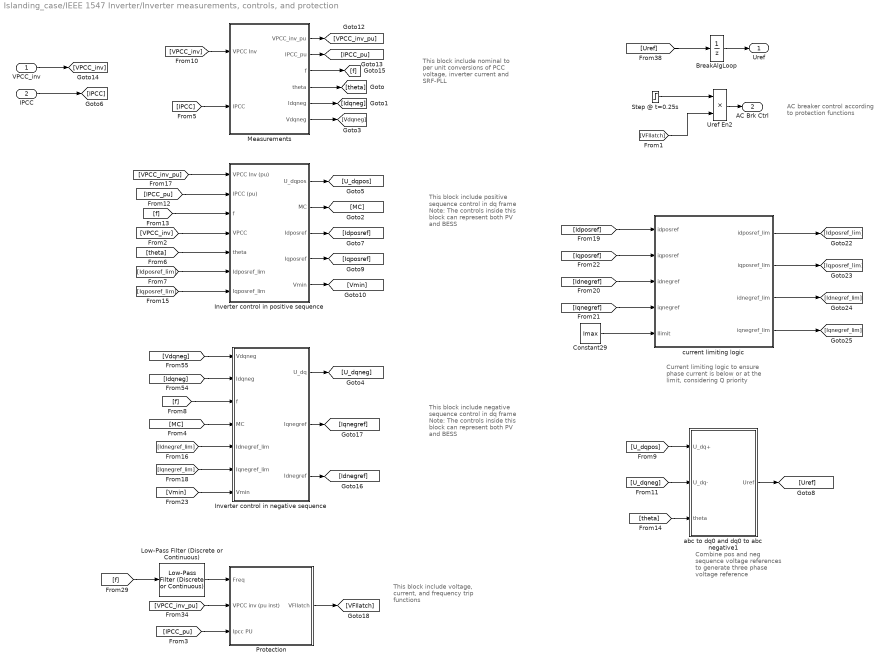
== system Islanding_case/IEEE 1547 Inverter/Inverter measurements, controls, and protection ==
  note: This block include negative sequence control in dq frame
      |
      | Note: The controls inside this block can represent both PV and BESS
  note: Current limiting logic to ensure phase current is below or at the limit, considering Q priority
  note: Combine pos and neg sequence voltage references to generate three phase voltage reference
  note: This block include voltage, current, and frequency trip functions
  note: This block include positive sequence control in dq frame
      |
      | Note: The controls inside this block can represent both PV and BESS
  note: This block include nominal to per unit conversions of PCC voltage, inverter current and SRF-PLL
  note: AC breaker control according to protection functions
  VPCC_inv : Inport
  IPCC : Inport  Port=2
  BreakAlgLoop : UnitDelay  SampleTime=Ts  HasFrameUpgradeWarning=on
  Constant29 : Constant  Value=Imax
  Inverter control in negative sequence : Subsystem  mask(DQ Regulator){Kpi=0.25, Kii=40, Kpv=12, Kiv=50, kd=0.175, L_dec=(RMSVnom*sqrt(3))^2/Pinv*0.2, En_Dec=0}
      mask prompts: Kpi "Current Proportional Gain (Kpi)"; Kii "Current Integral Gain (Kii)"; Kpv "Voltage Proportional Gain (Kpv)"; Kiv "Voltage Integral Gain (Kiv)"; kd "Decoupling Gain (kd)"; L_dec "Decoupling inductance (L_dec)"; En_Dec "Enable Decoupling (En_Dec) (1-Enabled, 0-Disabled)"
      mask help:
      | This block contains PI controllers that track the reference signal Idq_ref.
      | The PI gains are masked along with the decoupling gain kd.  DC voltage tracking
      | might also be implemented in this block.
      mask init:
      | if(En_Dec ~=1) %anything but 1 disables the decoupling
      |     En_Dec = 0;
      | end
  Inverter control in positive sequence : Subsystem
  Low-Pass Filter (Discrete or Continuous) : eeGeneralControl/Low-Pass Filter (Discrete or Continuous)  K=1  T=0.1  B=inf  A=-inf  init_option=Inherited from block input  x0=0  Ts=-1
  Measurements : Subsystem
  "Protection " : Subsystem
  Step @ t=0.25s : Step  Time=0.25  SampleTime=Ts
  Uref En2 : Product  RndMeth=Zero
  abc to dq0 and dq0 to abc negative1 : Subsystem
  current limiting logic : MATLAB Function  TreatAsAtomicUnit=on
  Uref : Outport  VectorParamsAs1DForOutWhenUnconnected=off
  AC Brk Ctrl : Outport  Port=2  VectorParamsAs1DForOutWhenUnconnected=off
  wires:
  [Vmin] -> Inverter control in negative sequence/7(Vmin)
  Inverter control in positive sequence/5(Vmin) -> [Vmin]
  [Iqnegref] -> current limiting logic/4(iqnegref)
  [Idnegref] -> current limiting logic/3(idnegref)
  [Iqposref] -> current limiting logic/2(iqposref)
  [Idposref] -> current limiting logic/1(idposref)
  Inverter control in negative sequence/3(Idnegref) -> [Idnegref]
  Inverter control in negative sequence/2(Iqnegref) -> [Iqnegref]
  Constant29/1 -> current limiting logic/5(Ilimit)
  current limiting logic/2(iqposref_lim) -> [Iqposref_lim]
  current limiting logic/3(idnegref_lim) -> [Idnegref_lim]
  current limiting logic/1(idposref_lim) -> [Idposref_lim]
  current limiting logic/4(iqnegref_lim) -> [Iqnegref_lim]
  [Iqnegref_lim] -> Inverter control in negative sequence/6(Iqnegref_lim)
  [Idnegref_lim] -> Inverter control in negative sequence/5(Idnegref_lim)
  Inverter control in positive sequence/4(Iqposref) -> [Iqposref]
  Inverter control in positive sequence/3(Idposref) -> [Idposref]
  [Iqposref_lim] -> Inverter control in positive sequence/7(Iqposref_lim)
  [Idposref_lim] -> Inverter control in positive sequence/6(Idposref_lim)
  [MC] -> Inverter control in negative sequence/4(MC)
  Inverter control in positive sequence/2(MC) -> [MC]
  [VFIlatch] -> Uref En2/2
  [theta] -> Inverter control in positive sequence/5(theta)
  Inverter control in positive sequence/1(U_dqpos) -> [U_dqpos]
  [theta] -> abc to dq0 and dq0 to abc negative1/3(theta)
  abc to dq0 and dq0 to abc negative1/1(Uref) -> [Uref]
  [U_dqneg] -> abc to dq0 and dq0 to abc negative1/2(U_dq-)
  [U_dqpos] -> abc to dq0 and dq0 to abc negative1/1(U_dq+)
  [Vdqneg] -> Inverter control in negative sequence/1(Vdqneg)
  Inverter control in negative sequence/1(U_dq) -> [U_dqneg]
  [f] -> Inverter control in negative sequence/3(f)
  [Idqneg] -> Inverter control in negative sequence/2(Idqneg)
  Measurements/6(Vdqneg) -> [Vdqneg]
  Measurements/5(Idqneg) -> [Idqneg]
  Measurements/4(theta) -> [theta]
  [IPCC_pu] -> "Protection "/3(Ipcc PU)
  [VPCC_inv] -> Inverter control in positive sequence/4(VPCC)
  Low-Pass Filter (Discrete or Continuous)/1 -> "Protection "/1(Freq)
  [Uref] -> BreakAlgLoop/1
  "Protection "/1(VFIlatch) -> [VFIlatch]
  [f] -> Low-Pass Filter (Discrete or Continuous)/1
  [VPCC_inv_pu] -> "Protection "/2(VPCC inv (pu inst))
  IPCC/1 -> [IPCC]
  VPCC_inv/1 -> [VPCC_inv]
  Step @ t=0.25s/1 -> Uref En2/1
  BreakAlgLoop/1 -> Uref/1
  Measurements/3(f) -> [f]
  Measurements/2(IPCC_pu) -> [IPCC_pu]
  Measurements/1(VPCC_inv_pu) -> [VPCC_inv_pu]
  [VPCC_inv_pu] -> Inverter control in positive sequence/1(VPCC Inv (pu))
  [IPCC] -> Measurements/2(IPCC)
  [VPCC_inv] -> Measurements/1(VPCC Inv)
  [f] -> Inverter control in positive sequence/3(f)
  [IPCC_pu] -> Inverter control in positive sequence/2(IPCC (pu))
  Uref En2/1 -> AC Brk Ctrl/1
